simulink model "sampleModel1457"  (R2023a)
settings: Solver=VariableStepAuto  StartTime=0.0  StopTime=10.0  RelTol=1e-3
libraries: hdlsllib x3, simulink x1
settings Model: Creator=user1  LastModifiedBy=user1

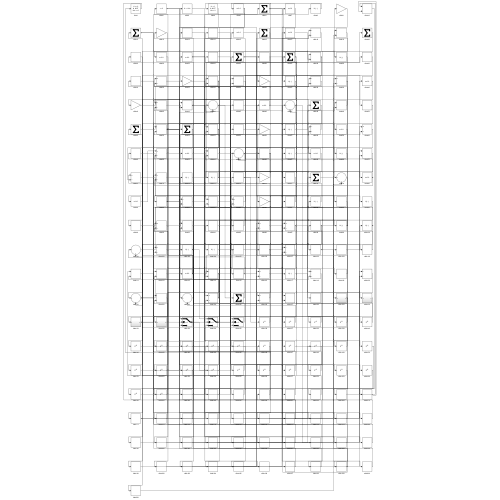
[thumbnail: Simulink's stored preview of the top-level diagram]
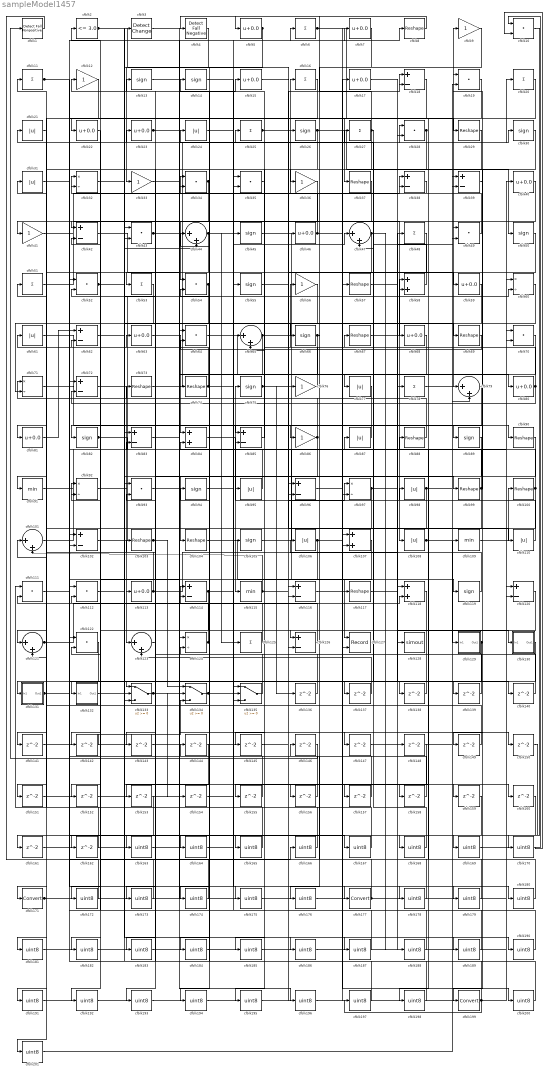
== system sampleModel1457 ==
  cfblk1 : hdlsllib/Logic and Bit Operations/Detect Fall Nonpositive  vinit=0  OutDataTypeStr=boolean
  cfblk{10,19,28,34..35,43,49,52,54,64,70,93,111..112,122} (15 alike) : DotProduct  OutDataTypeStr=Inherit: Inherit via internal rule
  cfblk{8,29,37,57,67,69,73..74,88,90,99..100,103..104,117} (15 alike) : Reshape
  cfblk{44,47,65,79,101,121,123} (7 alike) : Sum  Inputs=|++
  cfblk{18,38..39,42,62,72,83,85,96,102,114,116,120,126} (14 alike) : Sum  Inputs=+-
  cfblk{13..14,26,30,45,50,55,66,75,82,89,94,105,119} (14 alike) : Signum
  cfblk{21,24,31,61,77,87,95,98,106,108,110} (11 alike) : Abs  SaturateOnIntegerOverflow=off
  cfblk{58,84,107,118} (4 alike) : Sum
  cfblk109 : MinMax
  cfblk{6,11,16,20,25,27,48,51,53,78,125} (11 alike) : Sum  Inputs=+
  cfblk{5,7,15,17,22..23,40,46,59,63,68,80..81,113} (14 alike) : Bias  Bias=0.0  SaturateOnIntegerOverflow=off
  cfblk115 : MinMax
  cfblk{9,12,33,36,41,56,76,86} (8 alike) : Gain
  cfblk{32,60,71,92,97,124} (6 alike) : Product  Inputs=*/  RndMeth=Zero  SaturateOnIntegerOverflow=on
  cfblk127 : Record  FileSettingsInternal="{\"entries\":[{\"content\":{\"excelSettings\":{\"content\":{},\"type\":\"Streamout.ExcelSettings\"}},\"type\":\"Streamout.FileSettingStorage\",\"uuid\":\"\"}],\"packageUris\":[\"http:\\/\\/schema.mathworks.com\\/mf0\\/streamout_blocks\\/R2020a\"],\"version\":\"1.0\"}"  Layout=[1 1]  SignalsInternal="{\"entries\":[{\"content\":{\"signals\":[{\"content\":{\"blockPath\":[],\"dimensions\":[1],\"domain\":\"\",\"lineColor\":\"#a2142f\",\"plots\":[1],\"port\":1,\"sid\":[\"\"],\"signalID\":804,\"signalName\":\"cfblk104\"},\"type\":\"RecordBlkView.Signal\",\"uuid\":\"\"},{\"content\":{\"blockPath\":[],\"dimensions\":[1],\"domain\":\"\",\"lineColor\":\"#139fff\",\"plots\":[1],\"port\":2,\"sid\":[\"\"],\"signalID\":810,\"signalName\":\"cfblk9\"},\"type\":\"RecordBlkView.Signal\",\"uuid\":\"\"}]},\"type\":\"RecordBlkView.InputSignals\",\"uuid\":\"\"}],\"packageUris\":[\"http:\\/\\/schema.mathworks.com\\/mf0\\/streamout_blocks\\/R2020a\"],\"version\":\"1.0\"}"  VisualizationBindings="{\"xyplotplugin\":{\"info\":[{\"series\":[{\"bindingParametersList\":[{\"parameter\":\"X-Axis\",\"signalID\":804,\"signalName\":\"cfblk104\"},{\"parameter\":\"Y-Axis\",\"signalID\":810,\"signalName\":\"cfblk9\"}],\"seriesID\":53597}],\"subplotID\":1}]}}"  CompatibilityTag=XY  st=-1
  cfblk128 : ToWorkspace  VariableName=simout  SaveFormat=Timeseries  SampleTime=-1
  cfblk129 : Subsystem
      settings: LibrarySourceBlock=|
      | hdlsllib/Ports &
      | Subsystems/Subsystem
  cfblk130 : Subsystem
      settings: LibrarySourceBlock=|
      | hdlsllib/Ports &
      | Subsystems/Subsystem
  cfblk131 : Subsystem
      settings: LibrarySourceBlock=|
      | hdlsllib/Ports &
      | Subsystems/Subsystem
  cfblk132 : Subsystem
      settings: LibrarySourceBlock=|
      | hdlsllib/Ports &
      | Subsystems/Subsystem
  cfblk133 : Switch  SaturateOnIntegerOverflow=off  InputSameDT=off
  cfblk134 : Switch  SaturateOnIntegerOverflow=off  InputSameDT=off
  cfblk135 : Switch  SaturateOnIntegerOverflow=off  InputSameDT=off
  cfblk{136..162} (27 alike) : Delay  SampleTime=1
  cfblk{163..170,172..176,178..198,200..201} (36 alike) : DataTypeConversion  OutDataTypeStr=uint8  SaturateOnIntegerOverflow=off  RndMeth=Floor
  cfblk171 : DataTypeConversion  SaturateOnIntegerOverflow=off  RndMeth=Floor
  cfblk177 : DataTypeConversion  SaturateOnIntegerOverflow=off  RndMeth=Floor
  cfblk199 : DataTypeConversion  SaturateOnIntegerOverflow=off  RndMeth=Floor
  cfblk2 : hdlsllib/Logic and Bit Operations/Compare To Constant  relop=<=  const=3.0  OutDataTypeStr=boolean
  cfblk3 : simulink/Logic and Bit Operations/Detect Change  vinit=0  OutDataTypeStr=boolean
      settings: LibrarySourceBlock=|
      | hdlsllib/Logic and Bit
      | Operations/Detect
      | Change
  cfblk4 : hdlsllib/Logic and Bit Operations/Detect Fall Negative  vinit=0  OutDataTypeStr=boolean
  cfblk91 : MinMax
  wires:
  cfblk103/1 -> cfblk134/1, cfblk173/1
  cfblk45/1 -> cfblk119/1
  cfblk51/1 -> cfblk108/1
  cfblk81/1 -> cfblk62/1
  cfblk47/1 -> cfblk102/2, cfblk188/1
  cfblk108/1 -> cfblk129/1(In1), cfblk88/1
  cfblk105/1 -> cfblk87/1
  cfblk89/1 -> cfblk104/1
  cfblk67/1 -> cfblk58/1
  cfblk48/1 -> cfblk53/1
  cfblk110/1 -> cfblk75/1
  cfblk80/1 -> cfblk56/1, cfblk72/2
  cfblk135/1 -> cfblk12/1
  cfblk11/1 -> cfblk28/2, cfblk175/1
  cfblk86/1 -> cfblk32/1, cfblk153/1
  cfblk4/1 -> cfblk33/1
  cfblk12/1 -> cfblk22/1
  cfblk38/1 -> cfblk32/2
  cfblk61/1 -> cfblk85/1
  cfblk41/1 -> cfblk16/1
  cfblk125/1 -> cfblk94/1
  cfblk27/1 -> cfblk4/1, cfblk41/1, cfblk77/1
  cfblk55/1 -> cfblk38/1
  cfblk76/1 -> cfblk13/1
  cfblk63/1 -> cfblk84/1
  cfblk78/1 -> cfblk9/1
  cfblk7/1 -> cfblk36/1
  cfblk83/1 -> cfblk30/1
  cfblk39/1 -> cfblk199/1
  cfblk18/1 -> cfblk37/1
  cfblk87/1 -> cfblk86/1
  cfblk102/1 -> cfblk26/1
  cfblk72/1 -> cfblk123/1
  cfblk31/1 -> cfblk113/1
  cfblk6/1 -> cfblk29/1, cfblk200/1
  cfblk36/1 -> cfblk121/1
  cfblk73/1 -> cfblk20/1
  cfblk99/1 -> cfblk19/1, cfblk95/1, cfblk44/1, cfblk161/1
  cfblk97/1 -> cfblk133/1, cfblk130/1(In1)
  cfblk34/1 -> cfblk54/1, cfblk172/1
  cfblk124/1 -> cfblk71/1, cfblk92/2
  cfblk84/1 -> cfblk115/1
  cfblk66/1 -> cfblk155/1, cfblk156/1
  cfblk22/1 -> cfblk82/1
  cfblk8/1 -> cfblk5/1
  cfblk43/1 -> cfblk147/1, cfblk186/1
  cfblk123/1 -> cfblk73/1
  cfblk121/1 -> cfblk45/1, cfblk6/1
  cfblk13/1 -> cfblk69/1
  cfblk95/1 -> cfblk34/1
  cfblk104/1 -> cfblk127/1
  cfblk52/1 -> cfblk97/2, cfblk44/2, cfblk157/1, cfblk180/1
  cfblk24/1 -> cfblk55/1
  cfblk40/1 -> cfblk42/1
  cfblk2/1 -> cfblk76/1, cfblk114/2
  cfblk91/1 -> cfblk17/1
  cfblk82/1 -> cfblk85/2, cfblk58/2, cfblk62/2
  cfblk9/1 -> cfblk127/2
  cfblk74/1 -> cfblk60/2, cfblk61/1
  cfblk20/1 -> cfblk126/1
  cfblk100/1 -> cfblk27/1, cfblk149/1
  cfblk98/1 -> cfblk19/2, cfblk131/1(In1), cfblk133/3
  cfblk64/1 -> cfblk117/1
  cfblk109/1 -> cfblk100/1
  cfblk114/1 -> cfblk7/1, cfblk192/1
  cfblk88/1 -> cfblk11/1
  cfblk44/1 -> cfblk132/1(In1), cfblk125/1, cfblk160/1
  cfblk23/1 -> cfblk80/1, cfblk8/1
  cfblk49/1 -> cfblk2/1
  cfblk50/1 -> cfblk81/1
  cfblk132/1(Out1) -> cfblk38/2
  cfblk122/1 -> cfblk171/1
  cfblk69/1 -> cfblk64/2
  cfblk28/1 -> cfblk135/3, cfblk137/1
  cfblk62/1 -> cfblk3/1
  cfblk58/1 -> cfblk21/1
  cfblk26/1 -> cfblk50/1, cfblk105/1
  cfblk115/1 -> cfblk101/2, cfblk97/1
  cfblk25/1 -> cfblk90/1, cfblk18/2
  cfblk134/1 -> cfblk47/1, cfblk118/2, cfblk114/1
  cfblk65/1 -> cfblk128/1, cfblk110/1, cfblk135/2
  cfblk131/1(Out1) -> cfblk83/2, cfblk140/1
  cfblk71/1 -> cfblk89/1
  cfblk59/1 -> cfblk66/1
  cfblk113/1 -> cfblk48/1, cfblk51/1, cfblk92/1
  cfblk75/1 -> cfblk28/1, cfblk136/1
  cfblk21/1 -> cfblk121/2
  cfblk106/1 -> cfblk18/1, cfblk142/1
  cfblk119/1 -> cfblk106/1
  cfblk15/1 -> cfblk59/1
  cfblk42/1 -> cfblk124/1
  cfblk35/1 -> cfblk65/2
  cfblk126/1 -> cfblk103/1
  cfblk57/1 -> cfblk49/1
  cfblk92/1 -> cfblk79/2
  cfblk133/1 -> cfblk15/1, cfblk154/1
  cfblk32/1 -> cfblk68/1
  cfblk85/1 -> cfblk25/1
  cfblk17/1 -> cfblk118/1
  cfblk54/1 -> cfblk91/1, cfblk183/1
  cfblk14/1 -> cfblk177/1
  cfblk46/1 -> cfblk99/1, cfblk34/2
  cfblk101/1 -> cfblk40/1
  cfblk129/1(Out1) -> cfblk124/2, cfblk198/1
  cfblk56/1 -> cfblk71/2
  cfblk5/1 -> cfblk74/1, cfblk43/2
  cfblk136/1 -> cfblk84/2
  cfblk137/1 -> cfblk123/2
  cfblk19/1 -> cfblk138/1
  cfblk138/1 -> cfblk134/2
  cfblk117/1 -> cfblk139/1
  cfblk139/1 -> cfblk47/2
  cfblk140/1 -> cfblk52/2
  cfblk37/1 -> cfblk141/1
  cfblk141/1 -> cfblk126/2
  cfblk142/1 -> cfblk134/3
  cfblk29/1 -> cfblk143/1
  cfblk60/1 -> cfblk145/1
  cfblk146/1 -> cfblk1/1
  cfblk147/1 -> cfblk79/1
  cfblk149/1 -> cfblk101/1
  cfblk33/1 -> cfblk150/1
  cfblk16/1 -> cfblk151/1
  cfblk151/1 -> cfblk65/1
  cfblk77/1 -> cfblk152/1
  cfblk152/1 -> cfblk83/1
  cfblk154/1 -> cfblk54/2
  cfblk155/1 -> cfblk135/1
  cfblk156/1 -> cfblk133/2
  cfblk157/1 -> cfblk42/2
  cfblk130/1(Out1) -> cfblk158/1
  cfblk158/1 -> cfblk72/1
  cfblk94/1 -> cfblk159/1
  cfblk161/1 -> cfblk35/2
  cfblk53/1 -> cfblk162/1
  cfblk162/1 -> cfblk31/1
  cfblk144/1 -> cfblk163/1
  cfblk68/1 -> cfblk164/1
  cfblk164/1 -> cfblk144/1
  cfblk111/1 -> cfblk165/1
  cfblk165/1 -> cfblk63/1
  cfblk1/1 -> cfblk166/1
  cfblk166/1 -> cfblk111/1
  cfblk163/1 -> cfblk167/1
  cfblk167/1 -> cfblk111/2
  cfblk10/1 -> cfblk168/1
  cfblk168/1 -> cfblk67/1
  cfblk30/1 -> cfblk169/1
  cfblk169/1 -> cfblk10/1
  cfblk150/1 -> cfblk170/1
  cfblk170/1 -> cfblk10/2
  cfblk171/1 -> cfblk78/1, cfblk64/1
  cfblk172/1 -> cfblk122/1
  cfblk173/1 -> cfblk122/2
  cfblk70/1 -> cfblk174/1
  cfblk174/1 -> cfblk23/1
  cfblk175/1 -> cfblk70/1
  cfblk79/1 -> cfblk176/1
  cfblk176/1 -> cfblk70/2
  cfblk177/1 -> cfblk146/1, cfblk109/1, cfblk43/1
  cfblk3/1 -> cfblk178/1
  cfblk178/1 -> cfblk14/1
  cfblk96/1 -> cfblk179/1
  cfblk179/1 -> cfblk98/1
  cfblk180/1 -> cfblk96/1
  cfblk118/1 -> cfblk181/1
  cfblk181/1 -> cfblk96/2
  cfblk120/1 -> cfblk182/1
  cfblk182/1 -> cfblk57/1
  cfblk183/1 -> cfblk120/1
  cfblk160/1 -> cfblk184/1
  cfblk184/1 -> cfblk120/2
  cfblk148/1 -> cfblk185/1
  cfblk185/1 -> cfblk49/2
  cfblk186/1 -> cfblk148/1
  cfblk112/1 -> cfblk187/1
  cfblk187/1 -> cfblk35/1
  cfblk188/1 -> cfblk112/1
  cfblk143/1 -> cfblk189/1
  cfblk189/1 -> cfblk112/2
  cfblk116/1 -> cfblk190/1
  cfblk190/1 -> cfblk52/1
  cfblk159/1 -> cfblk191/1
  cfblk191/1 -> cfblk116/1
  cfblk192/1 -> cfblk116/2
  cfblk107/1 -> cfblk193/1
  cfblk193/1 -> cfblk46/1
  cfblk90/1 -> cfblk194/1
  cfblk194/1 -> cfblk107/1
  cfblk145/1 -> cfblk195/1
  cfblk195/1 -> cfblk107/2
  cfblk93/1 -> cfblk196/1
  cfblk196/1 -> cfblk60/1
  cfblk197/1 -> cfblk93/1
  cfblk198/1 -> cfblk93/2
  cfblk199/1 -> cfblk197/1, cfblk102/1, cfblk24/1
  cfblk200/1 -> cfblk39/1
  cfblk153/1 -> cfblk201/1
  cfblk201/1 -> cfblk39/2

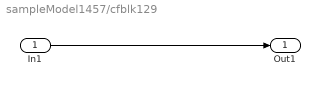
== system sampleModel1457/cfblk129 ==
  In1 : Inport
  Out1 : Outport
  wires:
  In1/1 -> Out1/1

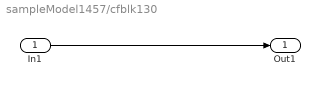
== system sampleModel1457/cfblk130 ==
  In1 : Inport
  Out1 : Outport
  wires:
  In1/1 -> Out1/1

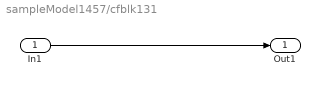
== system sampleModel1457/cfblk131 ==
  In1 : Inport
  Out1 : Outport
  wires:
  In1/1 -> Out1/1

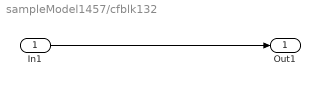
== system sampleModel1457/cfblk132 ==
  In1 : Inport
  Out1 : Outport
  wires:
  In1/1 -> Out1/1
